simulink library "wndlib1"  (Simulink 3.00)
libraries: fdctools x6
settings Model: LastModifiedBy=Dutchroll

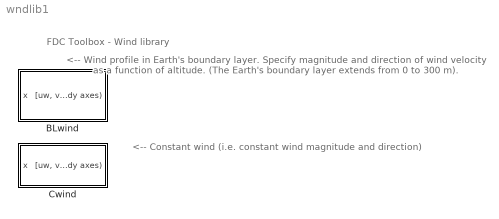
== system wndlib1 ==
  note: <-- Constant wind (i.e. constant wind magnitude and direction)
  note: FDC Toolbox - Wind library
  note: <-- Wind profile in Earth's boundary layer. Specify magnitude
      | and direction of wind velocity as a function of altitude.
      | (The Earth's boundary layer extends from 0 to 300 m).
  BLwind : Subsystem  mask(Windprofile in Earth's boundary layer){Vw=1*(u[1]^0.2545 - 0.4097)/1.3470, psi_w=180, theta_w=0}
      mask prompts: Vw "Wind speed function V(H) [m/s]:"; psi_w "Horizontal wind direction function, psi_w(H) [deg]:"; theta_w "Vertical  wind direction function, theta_w(H) [deg]:"
      mask help: Wind profile in Earth's boundary layer. Specify magnitude, horizontal direction and vertical direction as a function of the altitude (H). Input: state vector x, from the aircraft model. Output: [uw, vw, ww], resolved along aircraft's body-axes.
      mask init:
      | blockname = gcb;
      | Vwblock = [blockname, '/Vw [m//s]'];
      | psiblock = [blockname,'/psi_w [rad]'];
      | thetablock = [blockname,'/theta_w [rad]'];
      | 
      | set_param(Vwblock,'Expr',Vw);
      | set_param(psiblock,'Expr',[psi_w,'*pi/180']);
      | set_param(thetablock,'Expr',[theta_w,'*pi/180']);
      mask Help: eval('browse blwind')
      mask Display: disp('Windprofile in\nEarth''s boun-\ndary layer');
  Cwind : Subsystem  mask(Constant 3D wind vector){Vw=15, psi_w_deg=180, gamma_w_deg=0}
      mask prompts: Vw "Windspeed [m/s]:"; psi_w_deg "Horizontal wind direction [deg]:"; gamma_w_deg "Vertical  wind direction [deg]:"
      mask help: Constant wind vector. Specify wind velocity, horizontal wind direction, and vertical wind direction. Note: the horizontal wind direction equals zero when the wind is blowing FROM the North! The vertical wind direction is positive when blowing upwards.
      mask init:
      | psi_w = psi_w_deg * pi/180;
      | gamma_w = gamma_w_deg * pi/180;
      mask Help: eval('browse cwind')
      mask Display: disp('Constant\n3D wind vector')

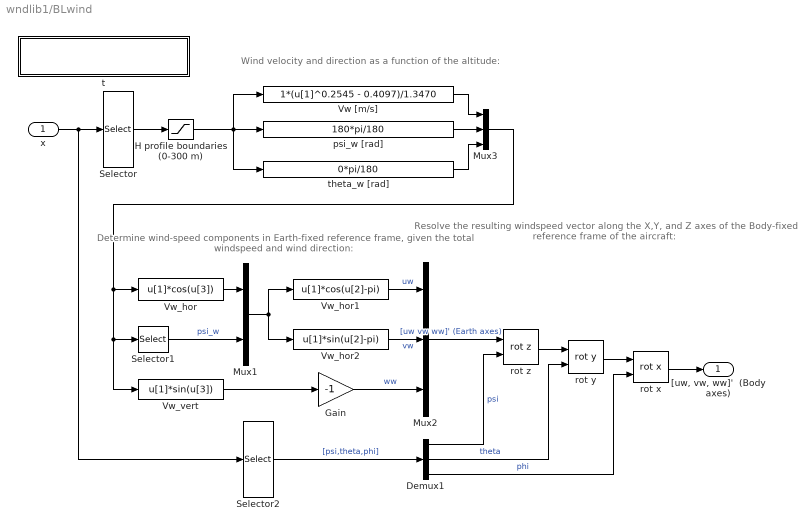
== system wndlib1/BLwind ==
  note: Determine wind-speed components in Earth-fixed reference
      | frame, given the total windspeed and wind direction:
  note: Resolve the resulting windspeed vector along the X,Y, and Z
      | axes of the Body-fixed reference frame of the aircraft:
  note: Wind velocity and direction as a function of the altitude:
  x : Inport  Port=1  PortWidth=-1  SampleTime=-1  DataType=auto
      settings: SignalType=auto
  Demux1 : Demux  Outputs=3
  Gain : Gain  Gain=-1  SaturateOnIntegerOverflow=on
  H profile boundaries (0-300 m) : Saturate  UpperLimit=300  LowerLimit=0
  Mux1 : Mux  Inputs=2
  Mux2 : Mux  Inputs=3
  Mux3 : Mux  Inputs=3
      settings: DisplayOption=none
  Selector : Selector  Elements=12  InputPortWidth=12
  Selector1 : Selector  Elements=2  InputPortWidth=3
  Selector2 : Selector  Elements=[7 8 9]  InputPortWidth=12
  Vw [m/s] : Fcn  Expr=1*(u[1]^0.2545 - 0.4097)/1.3470
  Vw_hor : Fcn  Expr=u[1]*cos(u[3])
  Vw_hor1 : Fcn  Expr=u[1]*cos(u[2]-pi)
  Vw_hor2 : Fcn  Expr=u[1]*sin(u[2]-pi)
  Vw_vert : Fcn  Expr=u[1]*sin(u[3])
  psi_w [rad] : Fcn  Expr=180*pi/180
  rot x : fdctools/rot x
  rot y : fdctools/rot y
  rot z : fdctools/rot z
  t : Subsystem
      settings: OpenFcn=browse blwind
      mask Display: disp('Wind profile in Earth''s boundary\nlayer. M.O. Rauw, March 2004')
  theta_w [rad] : Fcn  Expr=0*pi/180
  "[uw, vw, ww]'  (Body axes)" : Outport  Port=1
  wires:
  x/1 -> Selector/1, Selector2/1
  Mux2/1 -> rot z/1  "[uw vw ww]' (Earth axes)"
  Mux1/1 -> Vw_hor1/1, Vw_hor2/1
  Vw_hor2/1 -> Mux2/2  "vw"
  Vw_hor1/1 -> Mux2/1  "uw"
  Gain/1 -> Mux2/3  "ww"
  Vw_hor/1 -> Mux1/1
  Vw_vert/1 -> Gain/1
  rot x/1 -> "[uw, vw, ww]'  (Body axes)"/1
  rot z/1 -> rot y/1
  rot y/1 -> rot x/1
  Vw [m/s]/1 -> Mux3/1
  psi_w [rad]/1 -> Mux3/2
  theta_w [rad]/1 -> Mux3/3
  Mux3/1 -> Vw_hor/1, Vw_vert/1, Selector1/1
  H profile boundaries (0-300 m)/1 -> psi_w [rad]/1, Vw [m/s]/1, theta_w [rad]/1
  Selector/1 -> H profile boundaries (0-300 m)/1
  Selector1/1 -> Mux1/2  "psi_w"
  Demux1/1 -> rot z/2  "psi"
  Demux1/2 -> rot y/2  "theta"
  Demux1/3 -> rot x/2  "phi"
  Selector2/1 -> Demux1/1  "[psi,theta,phi]"

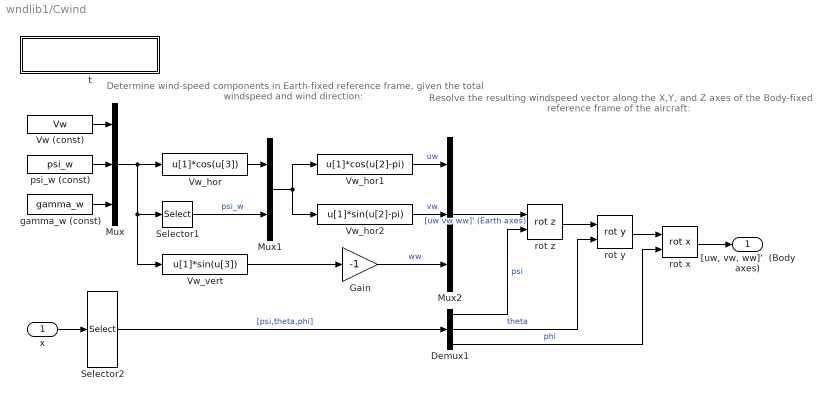
== system wndlib1/Cwind ==
  note: Resolve the resulting windspeed vector along the X,Y, and Z
      | axes of the Body-fixed reference frame of the aircraft:
  note: Determine wind-speed components in Earth-fixed reference
      | frame, given the total windspeed and wind direction:
  x : Inport  Port=1  PortWidth=-1  SampleTime=-1  DataType=auto
      settings: SignalType=auto
  Demux1 : Demux  Outputs=3
  Gain : Gain  Gain=-1  SaturateOnIntegerOverflow=on
  Mux : Mux  Inputs=3
      settings: DisplayOption=none
  Mux1 : Mux  Inputs=2
  Mux2 : Mux  Inputs=3
  Selector1 : Selector  Elements=2  InputPortWidth=3
  Selector2 : Selector  Elements=[7 8 9]  InputPortWidth=12
  Vw (const) : Constant  Value=Vw
  Vw_hor : Fcn  Expr=u[1]*cos(u[3])
  Vw_hor1 : Fcn  Expr=u[1]*cos(u[2]-pi)
  Vw_hor2 : Fcn  Expr=u[1]*sin(u[2]-pi)
  Vw_vert : Fcn  Expr=u[1]*sin(u[3])
  gamma_w (const) : Constant  Value=gamma_w
  psi_w (const) : Constant  Value=psi_w
  rot x : fdctools/rot x
  rot y : fdctools/rot y
  rot z : fdctools/rot z
  t : Subsystem
      settings: OpenFcn=browse cwind
      mask Display: disp('Constant wind vector\nM.O. Rauw, March 2004')
  "[uw, vw, ww]'  (Body axes)" : Outport  Port=1
  wires:
  rot x/1 -> "[uw, vw, ww]'  (Body axes)"/1
  Vw (const)/1 -> Mux/1
  gamma_w (const)/1 -> Mux/3
  psi_w (const)/1 -> Mux/2
  Mux/1 -> Vw_vert/1, Selector1/1, Vw_hor/1
  Vw_vert/1 -> Gain/1
  Vw_hor/1 -> Mux1/1
  Gain/1 -> Mux2/3  "ww"
  Vw_hor1/1 -> Mux2/1  "uw"
  Vw_hor2/1 -> Mux2/2  "vw"
  Mux1/1 -> Vw_hor2/1, Vw_hor1/1
  rot y/1 -> rot x/1
  rot z/1 -> rot y/1
  Mux2/1 -> rot z/1  "[uw vw ww]' (Earth axes)"
  Selector1/1 -> Mux1/2  "psi_w"
  Demux1/1 -> rot z/2  "psi"
  Demux1/2 -> rot y/2  "theta"
  Demux1/3 -> rot x/2  "phi"
  Selector2/1 -> Demux1/1  "[psi,theta,phi]"
  x/1 -> Selector2/1

== system wndlib1/BLwind/t ==

== system wndlib1/Cwind/t ==
